simulink model "modelo_AP_15"  (R2022b)
settings: Solver=VariableStepAuto  StartTime=0.0  StopTime=30  RelTol=1e-3
values from neighbouring files (symbols this model uses):
  FT_lat = FT_lat_function_elegante(p)    [SAS.m]
  K_deltaRbeta = -(F_beta - 1)*p.Cn_beta/p.Cn_deltaR    [Aumented_FT.m]    (also in SAS.m = -(F_beta_target - 1)*p.Cn_beta/p.Cn_deltaR)
  K_deltaRr = -(F_r - 1)*(p.Cn_r/p.Cn_deltaR)*(0.5*p.b/p.Us)    [Aumented_FT.m]    (also in SAS.m = -(F_r_target - 1)*(p.Cn_r/p.Cn_deltaR)*(0.5*p.b/p.Us))
  K_P_ = K_P(i)    [SAS.m]
libraries: cstblocks x7, simulink x1
settings Model: Creator=raulm  LastModifiedBy=abelu
settings ModelReferenceCC: EnableRefExpFcnMdlSchedulingChecks=on

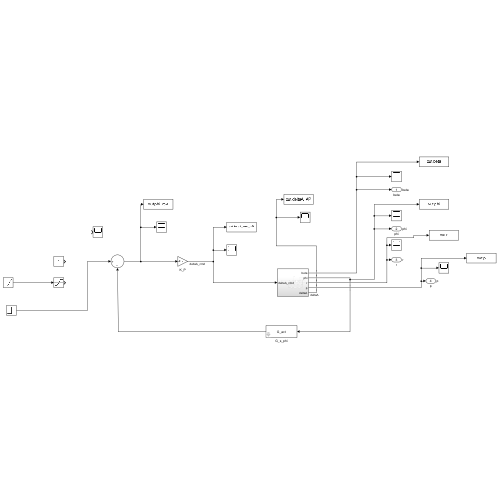
[thumbnail: Simulink's stored preview of the top-level diagram]
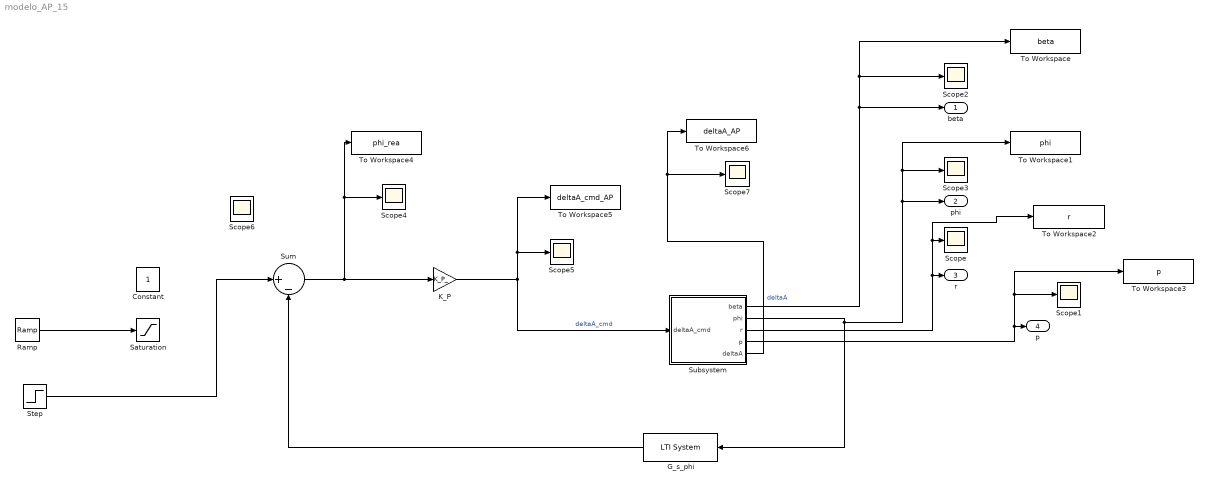
== system modelo_AP_15 ==
  Constant : Constant
  G_s_phi : cstblocks/LTI System  sys=G_act  IC=[]
  K_P : Gain  Gain=K_P_
  Ramp : simulink/Sources/Ramp  slope=1  start=0  InitialOutput=0
  Saturation : Saturate  UpperLimit=15  LowerLimit=0
  Scope{,1..7} (8 alike) : Scope
  Step : Step  SampleTime=0
  Subsystem : Subsystem
  Sum : Sum  Inputs=|+-
  To Workspace : ToWorkspace  VariableName=beta  SampleTime=-1
      settings: Save2DSignal=2-D array (concatenate along first dimension)
  To Workspace1 : ToWorkspace  VariableName=phi  SampleTime=-1
  To Workspace2 : ToWorkspace  VariableName=r  SampleTime=-1
  To Workspace3 : ToWorkspace  VariableName=p  SampleTime=-1
  To Workspace4 : ToWorkspace  VariableName=phi_rea  SampleTime=-1
      settings: Save2DSignal=2-D array (concatenate along first dimension)
  To Workspace5 : ToWorkspace  VariableName=deltaA_cmd_AP  SampleTime=-1
      settings: Save2DSignal=2-D array (concatenate along first dimension)
  To Workspace6 : ToWorkspace  VariableName=deltaA_AP  SampleTime=-1
      settings: Save2DSignal=2-D array (concatenate along first dimension)
  beta : Outport  SignalName=beta
  phi : Outport  Port=2  SignalName=phi
  r : Outport  Port=3  SignalName=r
  p : Outport  Port=4  SignalName=p
  wires:
  G_s_phi/1 -> Sum/2
  Sum/1 -> To Workspace4/1, Scope4/1, K_P/1
  Subsystem/4(p) -> To Workspace3/1, Scope1/1, p/1
  Subsystem/1(beta) -> To Workspace/1, Scope2/1, beta/1
  Subsystem/2(phi) -> G_s_phi/1, To Workspace1/1, Scope3/1, phi/1
  Subsystem/3(r) -> To Workspace2/1, Scope/1, r/1
  K_P/1 -> To Workspace5/1, Scope5/1, Subsystem/1(deltaA_cmd)  "deltaA_cmd"
  Ramp/1 -> Saturation/1
  Subsystem/5(deltaA) -> Scope7/1, To Workspace6/1  "deltaA"
  Step/1 -> Sum/1

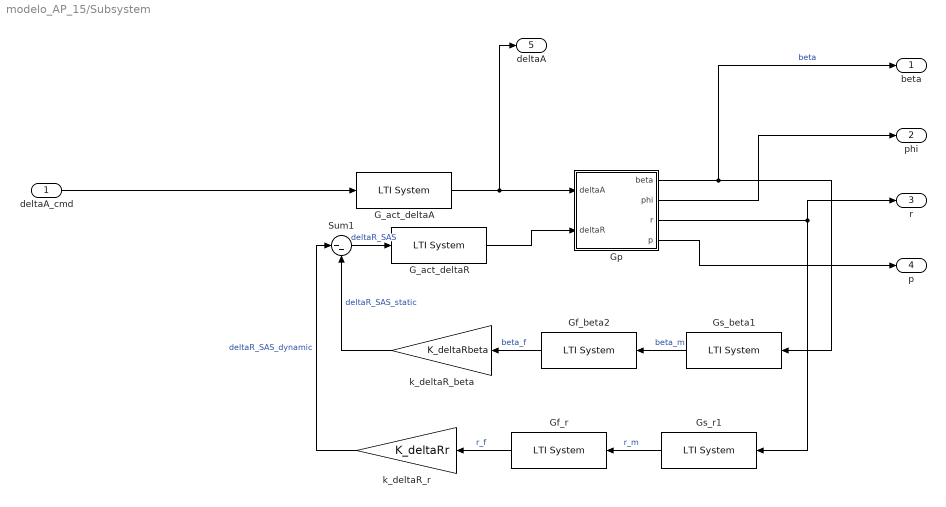
== system modelo_AP_15/Subsystem ==
  deltaA_cmd : Inport
  G_act_deltaA : cstblocks/LTI System  sys=G_act  IC=[]
  G_act_deltaR : cstblocks/LTI System  sys=G_act  IC=[]
  Gf_beta2 : cstblocks/LTI System  sys=1  IC=[]
  Gf_r : cstblocks/LTI System  sys=G_washout  IC=[]
  Gp : Subsystem
  Gs_beta1 : cstblocks/LTI System  sys=G_vane  IC=[]
  Gs_r1 : cstblocks/LTI System  sys=G_gyro  IC=[]
  Sum1 : Sum  Inputs=|--
  k_deltaR_beta : Gain  Gain=K_deltaRbeta
  k_deltaR_r : Gain  Gain=K_deltaRr
  beta : Outport
  phi : Outport  Port=2
  r : Outport  Port=3
  p : Outport  Port=4
  deltaA : Outport  Port=5
  wires:
  Gp/1(beta) -> beta/1, Gs_beta1/1  "beta"
  k_deltaR_beta/1 -> Sum1/2  "deltaR_SAS_static"
  G_act_deltaA/1 -> deltaA/1, Gp/1(deltaA)
  k_deltaR_r/1 -> Sum1/1  "deltaR_SAS_dynamic"
  Sum1/1 -> G_act_deltaR/1  "deltaR_SAS"
  Gs_beta1/1 -> Gf_beta2/1  "beta_m"
  Gp/3(r) -> Gs_r1/1, r/1
  Gf_beta2/1 -> k_deltaR_beta/1  "beta_f"
  Gs_r1/1 -> Gf_r/1  "r_m"
  G_act_deltaR/1 -> Gp/2(deltaR)
  Gp/4(p) -> p/1
  Gf_r/1 -> k_deltaR_r/1  "r_f"
  deltaA_cmd/1 -> G_act_deltaA/1
  Gp/2(phi) -> phi/1

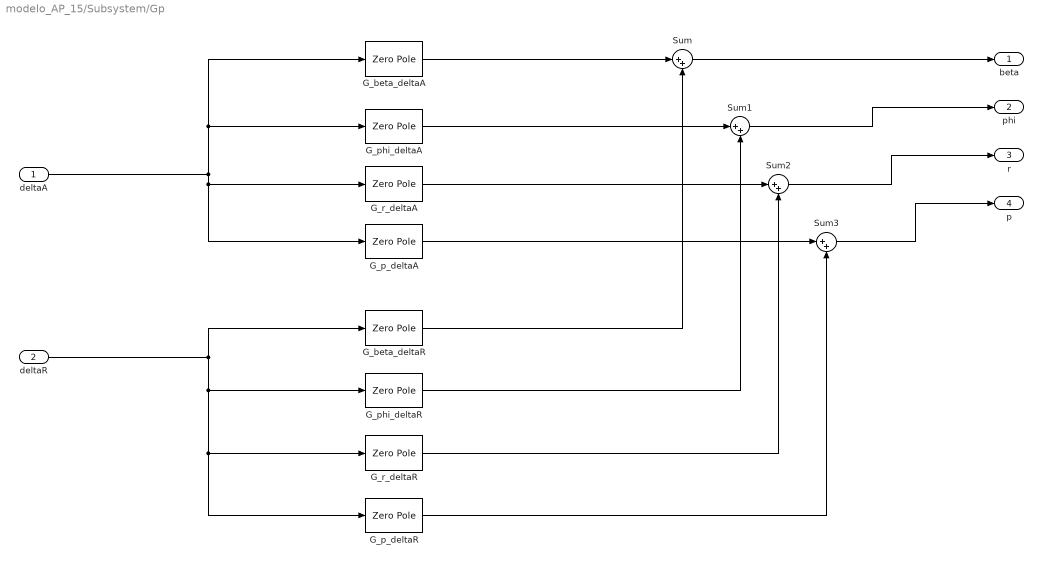
== system modelo_AP_15/Subsystem/Gp ==
  deltaA : Inport
  deltaR : Inport  Port=2
  G_beta_deltaA : ZeroPole  Zeros=FT_lat.fact.deltaA_beta.Z{1}  Poles=FT_lat.fact.deltaA_beta.P{1}  Gain=FT_lat.fact.deltaA_beta.K
  G_beta_deltaR : ZeroPole  Zeros=FT_lat.fact.deltaR_beta.Z{1}  Poles=FT_lat.fact.deltaR_beta.P{1}  Gain=FT_lat.fact.deltaR_beta.K
  G_p_deltaA : ZeroPole  Zeros=FT_lat.fact.deltaA_p.Z{1}  Poles=FT_lat.fact.deltaA_p.P{1}  Gain=FT_lat.fact.deltaA_p.K
  G_p_deltaR : ZeroPole  Zeros=FT_lat.fact.deltaR_p.Z{1}  Poles=FT_lat.fact.deltaR_p.P{1}  Gain=FT_lat.fact.deltaR_p.K
  G_phi_deltaA : ZeroPole  Zeros=FT_lat.fact.deltaA_phi.Z{1}  Poles=FT_lat.fact.deltaA_phi.P{1}  Gain=FT_lat.fact.deltaA_phi.K
  G_phi_deltaR : ZeroPole  Zeros=FT_lat.fact.deltaR_phi.Z{1}  Poles=FT_lat.fact.deltaR_phi.P{1}  Gain=FT_lat.fact.deltaR_phi.K
  G_r_deltaA : ZeroPole  Zeros=FT_lat.fact.deltaA_r.Z{1}  Poles=FT_lat.fact.deltaA_r.P{1}  Gain=FT_lat.fact.deltaA_r.K
  G_r_deltaR : ZeroPole  Zeros=FT_lat.fact.deltaR_r.Z{1}  Poles=FT_lat.fact.deltaR_r.P{1}  Gain=FT_lat.fact.deltaR_r.K
  Sum{,1..3} (4 alike) : Sum  Inputs=|++
  beta : Outport
  phi : Outport  Port=2
  r : Outport  Port=3
  p : Outport  Port=4
  wires:
  deltaR/1 -> G_p_deltaR/1, G_r_deltaR/1, G_phi_deltaR/1, G_beta_deltaR/1
  G_phi_deltaA/1 -> Sum1/1
  deltaA/1 -> G_p_deltaA/1, G_r_deltaA/1, G_phi_deltaA/1, G_beta_deltaA/1
  G_r_deltaR/1 -> Sum2/2
  G_p_deltaA/1 -> Sum3/1
  G_r_deltaA/1 -> Sum2/1
  G_beta_deltaR/1 -> Sum/2
  Sum2/1 -> r/1
  Sum3/1 -> p/1
  Sum/1 -> beta/1
  G_p_deltaR/1 -> Sum3/2
  Sum1/1 -> phi/1
  G_beta_deltaA/1 -> Sum/1
  G_phi_deltaR/1 -> Sum1/2
